simulink model "VehicleDynamics"  (R2022a)
settings: Solver=VariableStepAuto  StartTime=0.0  StopTime=t_end_sim  FixedStep=dt_sim  RelTol=1e-3  EnableMultiTasking=on
values from neighbouring files (symbols this model uses):
  A_sim = [(-CF-CR)/(m*Vv),(-CF*a+CR*b-m*Vv^2)/(m*Vv^2) ... (first row only)    [Dynamics.m]
  ay_max = 8    [Dynamics.m]
  B_sim = [CF/(m*Vv) -CR/(m*Vv) ... (first row only)    [Dynamics.m]
  beta_max = 10    [Dynamics.m]
  C_sim = [1,0 ... (first row only)    [Dynamics.m]
  D_sim = [0 0 ... (first row only)    [Dynamics.m]
  delta_vol_max_ramp = 200    [Dynamics.m]
  dvol_max = 10    [Dynamics.m]
  L = 2.85    [Dynamics.m]
  sel_man = 1    [Dynamics.m]
  t_end_sim = 45    [Dynamics.m]
  tau_s = 15    [Dynamics.m]
  V = V/3.6    (= 27.7777777778)    [Dynamics.m]
libraries: simulink_extras x6, simulink x5
settings Model: Creator=gianl  LastModifiedBy=Vincentiu_Mocanu
settings SolverCC: AlgebraicLoopSolver=TrustRegion
settings DataIOCC: ReturnWorkspaceOutputs=off  ReturnWorkspaceOutputsName=out_SLX
settings OptimizationCC: LifeSpan=1
settings DebuggingCC: UnconnectedInputMsg=warning  UnconnectedOutputMsg=warning  UnconnectedLineMsg=warning  SFExecutionAtInitializationDiag=none  SFMachineParentedDataDiag=warning  ArithmeticOperatorsInVariantConditions=warning
settings SFSimCC: SimUseLocalCustomCode=off  CustomCodeUndefinedFunction=UseInterfaceOnly
settings RTWCC: RTWUseLocalCustomCode=off  DLArmComputeVersion=19.05
settings CodeAppCC: StateflowObjectComments=on

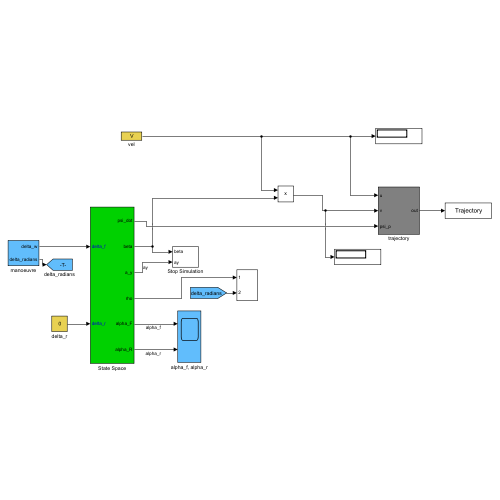
[thumbnail: Simulink's stored preview of the top-level diagram]
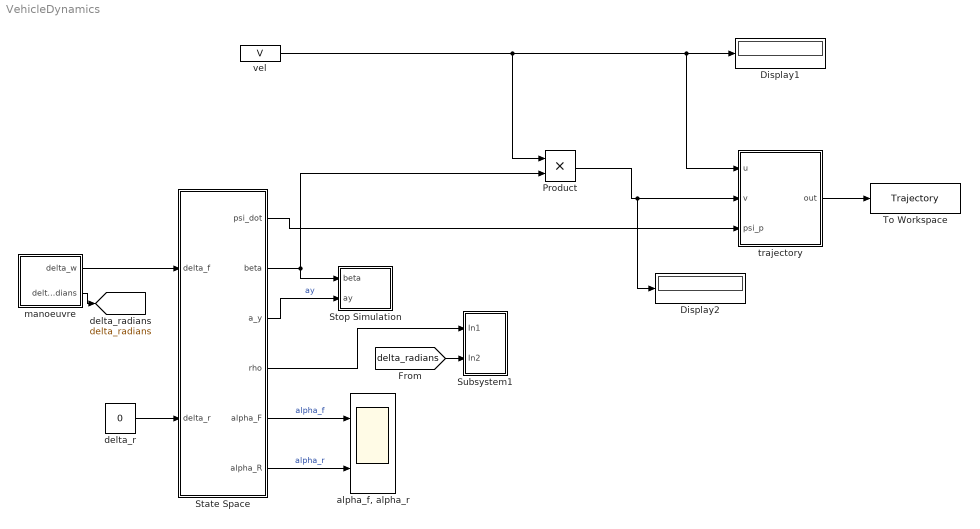
== system VehicleDynamics ==
  Display1 : Display
  Display2 : Display
  Product : Product
  State Space : Subsystem
  Stop Simulation : Subsystem
  Subsystem1 : Subsystem
  To Workspace : ToWorkspace  VariableName=Trajectory  SaveFormat=Timeseries  SampleTime=-1
  "alpha_f, alpha_r" : Scope  NumInputPorts=2
  delta_r : Constant  Value=0
  manoeuvre : Subsystem
  trajectory : Subsystem
  vel : Constant  Value=V
  tag scope: delta_radians=global
  wires:
  manoeuvre/1(delta_w) -> State Space/1(delta_f)
  vel/1 -> Product/1, Display1/1, trajectory/1(u)
  delta_r/1 -> State Space/2(delta_r)
  State Space/5(alpha_F) -> "alpha_f, alpha_r"/1  "alpha_f"
  State Space/6(alpha_R) -> "alpha_f, alpha_r"/2  "alpha_r"
  State Space/4(rho) -> Subsystem1/1(In1)
  State Space/3(a_y) -> Stop Simulation/2(ay)  "ay"
  manoeuvre/2(delta_radians) -> [delta_radians]
  State Space/1(psi_dot) -> trajectory/3(psi_p)
  State Space/2(beta) -> Stop Simulation/1(beta), Product/2
  trajectory/1(out) -> To Workspace/1
  [delta_radians] -> Subsystem1/2(In2)
  Product/1 -> Display2/1, trajectory/2(v)

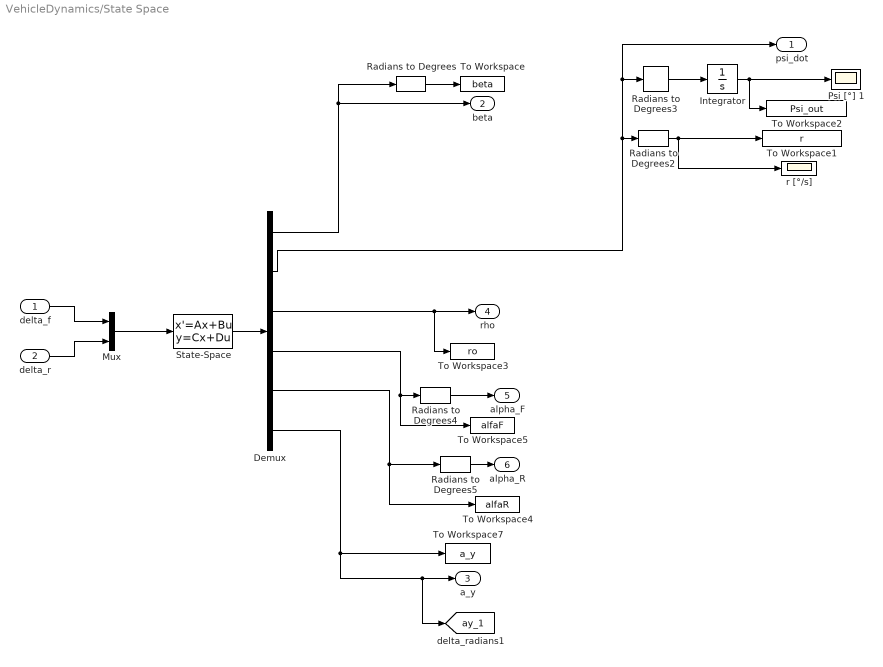
== system VehicleDynamics/State Space ==
  delta_f : Inport
  delta_r : Inport  Port=2
  Demux : Demux  Outputs=6
  Integrator : Integrator
  Mux : Mux  Inputs=2
  Psi [°] 1 : Scope
  Radians to Degrees{,2..5} (5 alike) : simulink_extras/Transformations/Radians to Degrees
  State-Space : StateSpace  A=A_sim  B=B_sim  C=C_sim  D=D_sim  InitialCondition=[0 0]  ContinuousStateAttributes={'sideslip_angle','yaw_rate'}
  To Workspace : ToWorkspace  VariableName=beta  SaveFormat=Timeseries  SampleTime=-1
  To Workspace1 : ToWorkspace  VariableName=r  SaveFormat=Timeseries  SampleTime=-1
  To Workspace2 : ToWorkspace  VariableName=Psi_out  SaveFormat=Timeseries  SampleTime=-1
  To Workspace3 : ToWorkspace  VariableName=ro  SaveFormat=Timeseries  SampleTime=-1
  To Workspace4 : ToWorkspace  VariableName=alfaR  SaveFormat=Timeseries  SampleTime=-1
  To Workspace5 : ToWorkspace  VariableName=alfaF  SaveFormat=Timeseries  SampleTime=-1
  To Workspace7 : ToWorkspace  VariableName=a_y  SaveFormat=Timeseries  SampleTime=-1
      settings: Save2DSignal=2-D array (concatenate along first dimension)
  r [°/s] : Scope
  psi_dot : Outport  VectorParamsAs1DForOutWhenUnconnected=off
  beta : Outport  Port=2  VectorParamsAs1DForOutWhenUnconnected=off
  a_y : Outport  Port=3  VectorParamsAs1DForOutWhenUnconnected=off
  rho : Outport  Port=4  VectorParamsAs1DForOutWhenUnconnected=off
  alpha_F : Outport  Port=5  VectorParamsAs1DForOutWhenUnconnected=off
  alpha_R : Outport  Port=6  VectorParamsAs1DForOutWhenUnconnected=off
  tag scope: ay_1=global
  wires:
  Demux/2 -> psi_dot/1, Radians to Degrees3/1, Radians to Degrees2/1
  Demux/1 -> Radians to Degrees/1, beta/1
  State-Space/1 -> Demux/1
  Radians to Degrees/1 -> To Workspace/1
  Radians to Degrees2/1 -> r [°/s]/1, To Workspace1/1
  Demux/3 -> rho/1, To Workspace3/1
  Demux/4 -> Radians to Degrees4/1, To Workspace5/1
  Demux/5 -> Radians to Degrees5/1, To Workspace4/1
  Radians to Degrees3/1 -> Integrator/1
  Integrator/1 -> To Workspace2/1, Psi [°] 1/1
  delta_f/1 -> Mux/1
  Mux/1 -> State-Space/1
  delta_r/1 -> Mux/2
  Demux/6 -> [ay_1], a_y/1, To Workspace7/1
  Radians to Degrees4/1 -> alpha_F/1
  Radians to Degrees5/1 -> alpha_R/1

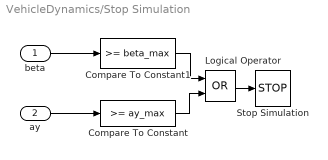
== system VehicleDynamics/Stop Simulation ==
  beta : Inport
  ay : Inport  Port=2
  Compare To Constant : simulink/Logic and Bit Operations/Compare To Constant  relop=>=  const=ay_max  OutDataTypeStr=boolean
  Compare To Constant1 : simulink/Logic and Bit Operations/Compare To Constant  relop=>=  const=beta_max  OutDataTypeStr=boolean
  Logical Operator : Logic  Operator=OR  AllPortsSameDT=off  OutDataTypeStr=boolean
  Stop Simulation : Stop
  wires:
  Logical Operator/1 -> Stop Simulation/1
  ay/1 -> Compare To Constant/1
  beta/1 -> Compare To Constant1/1
  Compare To Constant/1 -> Logical Operator/2
  Compare To Constant1/1 -> Logical Operator/1

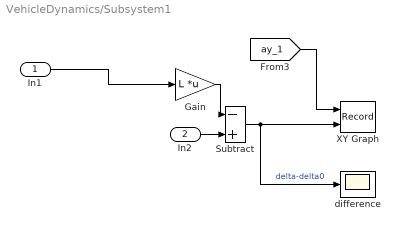
== system VehicleDynamics/Subsystem1 ==
  In1 : Inport
  In2 : Inport  Port=2
  Gain : Gain  Gain=L  Multiplication=Matrix(K*u)
  Subtract : Sum  Inputs=-+
  XY Graph : Record  FileSettingsInternal="{\"entries\":[{\"content\":{\"excelSettings\":{\"content\":{},\"type\":\"Streamout.ExcelSettings\"}},\"type\":\"Streamout.FileSettingStorage\",\"uuid\":\"d3249077-0703-4b87-aced-a8f336e08e20\"}],\"packageUris\":[\"http://schema.mathworks.com/mf0/streamout_blocks/R2020a\"],\"version\":\"1.0\"}"  Layout=[1 1]  SignalsInternal="{\"entries\":[{\"content\":{\"signals\":[{\"content\":{\"blockPath\":[\"VehicleDynamics/Subsystem1/XY Graph\"],\"channel\":[],\"dimensions\":[1],\"domain\":\"VehicleDynamics/Subsystem1/XY Graph\",\"lineColor\":\"#77ac30\",\"plots\":[],\"port\":1,\"sid\":[],\"signalID\":119,\"signalName\":\"From3\"},\"type\":\"RecordBlkView.Signal\",\"uuid\":\"79ecad71-6918-4463-9e88-4dc9082c1bb4\"},{\"content\":{\"blockPath\":[\"VehicleDynamics/Subsystem1/XY Graph\"],\"channel\":[],\"dimensions\":[1],\"domain\":\"VehicleDynamics/Subsystem1/XY Graph\",\"lineColor\":\"#4dbeee\",\"plots\":[],\"port\":2,\"sid\":[],\"signalID\":122,\"signalName\":\"delta-delta0\"},\"type\":\"RecordBlkView.Signal\",\"uuid\":\"8d7844a4-fd70-4fea-a8ef-3c2e6f74f73d\"}]},\"type\":\"RecordBlkView.InputSignals\",\"uuid\":\"e66ac0a6-40b9-4b32-a008-8d59b009c7a9\"}],\"packageUris\":[\"http://schema.mathworks.com/mf0/streamout_blocks/R2020a\"],\"version\":\"1.0\"}"  VisualizationBindings="{\"xyplotplugin\":{\"info\":[{\"series\":[],\"subplotID\":1}]}}"  CompatibilityTag=XY
  difference : Scope
  wires:
  Subtract/1 -> difference/1, XY Graph/2  "delta-delta0"
  In2/1 -> Subtract/2
  Gain/1 -> Subtract/1
  [ay_1] -> XY Graph/1
  In1/1 -> Gain/1

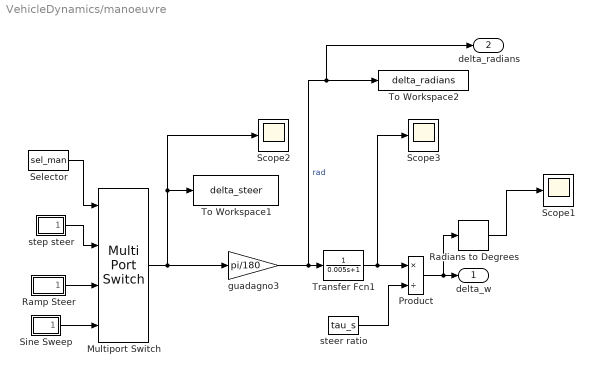
== system VehicleDynamics/manoeuvre ==
  Multiport Switch : MultiPortSwitch  SaturateOnIntegerOverflow=off  InputSameDT=off
  Product : Product  Inputs=*/  RndMeth=Zero
  Radians to Degrees : simulink_extras/Transformations/Radians to Degrees
  Ramp Steer : Subsystem
  Scope1 : Scope
  Scope2 : Scope
  Scope3 : Scope
  Selector : Constant  Value=sel_man
  Sine Sweep : Subsystem
  To Workspace1 : ToWorkspace  VariableName=delta_steer  SaveFormat=Timeseries  SampleTime=-1
  To Workspace2 : ToWorkspace  VariableName=delta_radians  SaveFormat=Timeseries  SampleTime=-1
  Transfer Fcn1 : TransferFcn  Denominator=[0.005 1]
  guadagno3 : Gain  Gain=pi/180  SaturateOnIntegerOverflow=on  OutDataTypeStr=Inherit: Same as input  ParamDataTypeStr=Inherit: Same as input
  "steer ratio " : Constant  Value=tau_s
  step steer : Subsystem
  delta_w : Outport  VectorParamsAs1DForOutWhenUnconnected=off
  delta_radians : Outport  Port=2  VectorParamsAs1DForOutWhenUnconnected=off
  wires:
  Selector/1 -> Multiport Switch/1
  Ramp Steer/1(delta) -> Multiport Switch/3
  step steer/1(delta) -> Multiport Switch/2
  Multiport Switch/1 -> To Workspace1/1, Scope2/1, guadagno3/1
  guadagno3/1 -> delta_radians/1, To Workspace2/1, Transfer Fcn1/1  "rad"
  "steer ratio "/1 -> Product/2
  Product/1 -> Radians to Degrees/1, delta_w/1
  Transfer Fcn1/1 -> Scope3/1, Product/1
  Radians to Degrees/1 -> Scope1/1
  Sine Sweep/1(delta) -> Multiport Switch/4

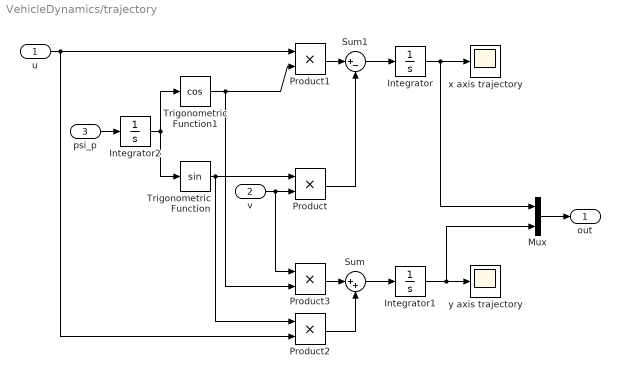
== system VehicleDynamics/trajectory ==
  u : Inport
  v : Inport  Port=2
  psi_p : Inport  Port=3
  Integrator : Integrator
  Integrator1 : Integrator
  Integrator2 : Integrator
  Mux : Mux  Inputs=2
  Product{,1..3} (4 alike) : Product  InputSameDT=on  SaturateOnIntegerOverflow=on  OutDataTypeStr=Inherit: Same as first input
  Sum : Sum  Inputs=|++  InputSameDT=on  SaturateOnIntegerOverflow=on  OutDataTypeStr=Inherit: Same as first input
  Sum1 : Sum  Inputs=|+-  InputSameDT=on  SaturateOnIntegerOverflow=on  OutDataTypeStr=Inherit: Same as first input
  Trigonometric Function : Trigonometry
  Trigonometric Function1 : Trigonometry  Operator=cos
  x axis trajectory : Scope
  y axis trajectory : Scope
  out : Outport
  wires:
  psi_p/1 -> Integrator2/1
  Product1/1 -> Sum1/1
  Product/1 -> Sum1/2
  Sum1/1 -> Integrator/1
  Trigonometric Function/1 -> Product/1, Product2/1
  u/1 -> Product2/2, Product1/1
  v/1 -> Product/2, Product3/1
  Trigonometric Function1/1 -> Product1/2, Product3/2
  Product3/1 -> Sum/1
  Product2/1 -> Sum/2
  Sum/1 -> Integrator1/1
  Integrator/1 -> Mux/1, x axis trajectory/1
  Integrator2/1 -> Trigonometric Function/1, Trigonometric Function1/1
  Integrator1/1 -> Mux/2, y axis trajectory/1
  Mux/1 -> out/1

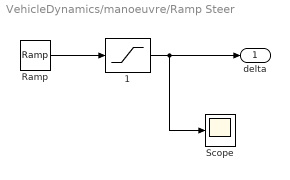
== system VehicleDynamics/manoeuvre/Ramp Steer ==
  "  1" : Saturate  UpperLimit=delta_vol_max_ramp  LowerLimit=-delta_vol_max_ramp
  Ramp : simulink/Sources/Ramp  slope=10  start=1  InitialOutput=0
  Scope : Scope
  delta : Outport  VectorParamsAs1DForOutWhenUnconnected=off
  wires:
  Ramp/1 -> "  1"/1
  "  1"/1 -> Scope/1, delta/1

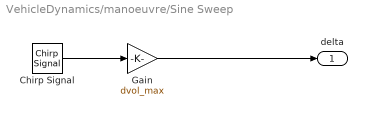
== system VehicleDynamics/manoeuvre/Sine Sweep ==
  Chirp Signal : simulink/Sources/Chirp Signal  f1=0.01  T=t_end_sim  f2=freq
  Gain : Gain  Gain=dvol_max
  delta : Outport  InitialOutput=0  VectorParamsAs1DForOutWhenUnconnected=off
  wires:
  Chirp Signal/1 -> Gain/1
  Gain/1 -> delta/1

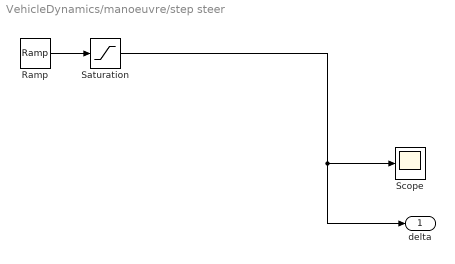
== system VehicleDynamics/manoeuvre/step steer ==
  Ramp : simulink/Sources/Ramp  slope=400  start=1  InitialOutput=0
  Saturation : Saturate  UpperLimit=dvol_max  LowerLimit=0
  Scope : Scope
  delta : Outport  VectorParamsAs1DForOutWhenUnconnected=off
  wires:
  Ramp/1 -> Saturation/1
  Saturation/1 -> delta/1, Scope/1
